simulink model "quadcopter_pd_test"  (R2015b)
settings: Solver=VariableStepAuto  StartTime=0.0  StopTime=50  RelTol=1e-3
undefined symbols (not defined in the file): omegalim, seed
libraries: vrlib x2
settings Model: Creator=Daniel  LastModifiedBy=mgreiff

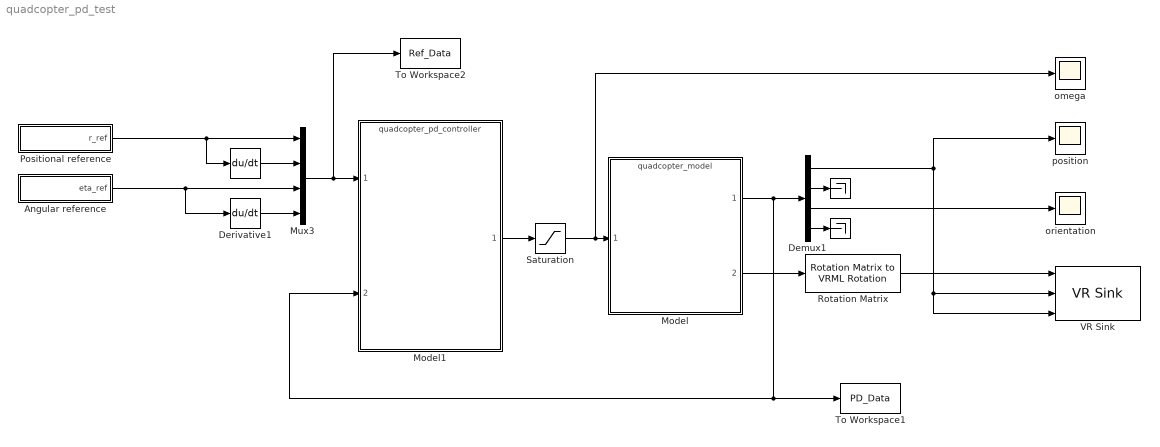
== system quadcopter_pd_test ==
  "  " : Terminator
  "   " : Terminator
  "        " : Derivative
  Angular reference : Subsystem
  Demux1 : Demux  Outputs=[3,3,3,3]
  Derivative1 : Derivative
  Model : ModelReference  ModelNameDialog=quadcopter_model.mdl  SimulationMode=Normal  ModelReferenceVersion=1.117  CopyOfModelName=quadcopter_model.mdl
  Model1 : ModelReference  ModelNameDialog=quadcopter_pd_controller.mdl  SimulationMode=Normal  ModelReferenceVersion=1.67  CopyOfModelName=quadcopter_pd_controller.mdl
  Mux3 : Mux  Inputs=[3,3,3,3]
  Positional reference : Subsystem
  Rotation Matrix : vrlib/Utilities/Rotation Matrix to VRML Rotation  maxzero=1e-12
  Saturation : Saturate  UpperLimit=omegalim(2)  LowerLimit=omegalim(1)
  To Workspace1 : ToWorkspace  VariableName=PD_Data  SaveFormat=Timeseries  SampleTime=-1
  To Workspace2 : ToWorkspace  VariableName=Ref_Data  SaveFormat=Timeseries  SampleTime=-1
  VR Sink : vrlib/VR Sink  InstantiateOnLoad=on  SampleTime=0.1  ViewEnable=on  RemoteChange=off  RemoteView=off  FieldsWritten=copter.rotation.4.1.1.double#copter.translation.3.1.1.double#vp.translation.3.1.1.double  WorldFileName=copter_world.wrl  WorldDescription=quadcopter_world  AutoView=on  VideoDimensions=[]  AllowVariableSize=off
  "omega " : Scope
  orientation : Scope
  position : Scope
  wires:
  Rotation Matrix/1 -> VR Sink/1
  Model1/1 -> Saturation/1
  Saturation/1 -> Model/1, "omega "/1
  Model/2 -> Rotation Matrix/1
  Demux1/2 -> "  "/1
  Demux1/4 -> "   "/1
  Demux1/1 -> VR Sink/3, VR Sink/2, position/1
  Demux1/3 -> orientation/1
  Angular reference/1(eta_ref) -> Derivative1/1, Mux3/3
  Positional reference/1(r_ref) -> Mux3/1, "        "/1
  "        "/1 -> Mux3/2
  Derivative1/1 -> Mux3/4
  Model/1 -> To Workspace1/1, Model1/2, Demux1/1
  Mux3/1 -> To Workspace2/1, Model1/1

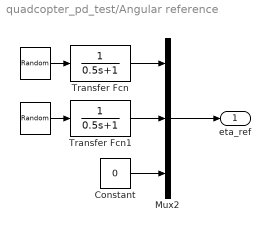
== system quadcopter_pd_test/Angular reference ==
  " " : UniformRandomNumber  Minimum=-0.2  Maximum=0.2  Seed=4+seed  SampleTime=10
  "   " : UniformRandomNumber  Minimum=-0.2  Maximum=0.2  Seed=3+seed  SampleTime=10
  Constant : Constant  Value=0
  Mux2 : Mux  Inputs=3
  Transfer Fcn : TransferFcn  Denominator=[0.5 1]
  Transfer Fcn1 : TransferFcn  Denominator=[0.5 1]
  eta_ref : Outport
  wires:
  Mux2/1 -> eta_ref/1
  "   "/1 -> Transfer Fcn/1
  " "/1 -> Transfer Fcn1/1
  Transfer Fcn/1 -> Mux2/1
  Transfer Fcn1/1 -> Mux2/2
  Constant/1 -> Mux2/3

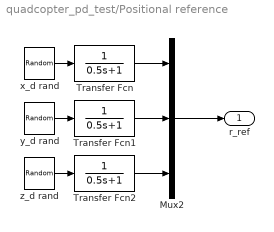
== system quadcopter_pd_test/Positional reference ==
  Mux2 : Mux  Inputs=3
  Transfer Fcn : TransferFcn  Denominator=[0.5 1]
  Transfer Fcn1 : TransferFcn  Denominator=[0.5 1]
  Transfer Fcn2 : TransferFcn  Denominator=[0.5 1]
  x_d rand : UniformRandomNumber  Minimum=-30  Maximum=30  Seed=0+seed  SampleTime=10
  y_d rand : UniformRandomNumber  Minimum=-30  Maximum=30  Seed=1+seed  SampleTime=10
  z_d rand : UniformRandomNumber  Minimum=0  Maximum=15  Seed=2+seed  SampleTime=10
  r_ref : Outport
  wires:
  Mux2/1 -> r_ref/1
  x_d rand/1 -> Transfer Fcn/1
  y_d rand/1 -> Transfer Fcn1/1
  z_d rand/1 -> Transfer Fcn2/1
  Transfer Fcn/1 -> Mux2/1
  Transfer Fcn1/1 -> Mux2/2
  Transfer Fcn2/1 -> Mux2/3
